simulink model "van_der_pol"  (R2015a)
settings: Solver=ode45  StartTime=0.0  StopTime=10.0  RelTol=1e-3
values from neighbouring files (symbols this model uses):
  mu = 5    [main.m]
undefined symbols (not defined in the file or in its folder): x_1, x_2
settings Model: Creator=Martin  LastModifiedBy=Martin

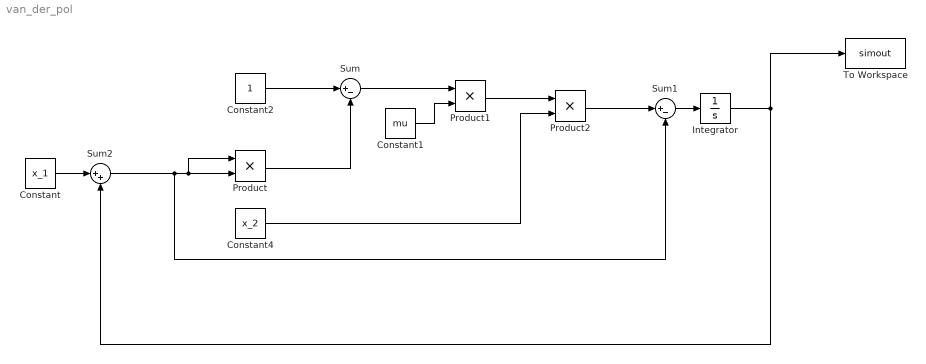
== system van_der_pol ==
  Constant : Constant  Value=x_1
  Constant1 : Constant  Value=mu
  Constant2 : Constant
  Constant4 : Constant  Value=x_2
  Integrator : Integrator
  Product : Product
  Product1 : Product
  Product2 : Product
  Sum : Sum  Inputs=|+-
  Sum1 : Sum  Inputs=|+-
  Sum2 : Sum  Inputs=|++
  To Workspace : ToWorkspace  VariableName=simout  SaveFormat=Timeseries  SampleTime=-1
  wires:
  Sum2/1 -> Sum1/2, Product/1, Product/2
  Constant2/1 -> Sum/1
  Product/1 -> Sum/2
  Sum/1 -> Product1/1
  Constant1/1 -> Product1/2
  Product1/1 -> Product2/1
  Constant4/1 -> Product2/2
  Product2/1 -> Sum1/1
  Integrator/1 -> To Workspace/1, Sum2/2
  Constant/1 -> Sum2/1
  Sum1/1 -> Integrator/1
